simulink model "NaoLinearidadeAtuador"  (R2023b)
settings: Solver=FixedStepAuto  StartTime=0.0  StopTime=tf  FixedStep=step_modelo  RelTol=1e-3
values from neighbouring files (symbols this model uses):
  actuator_nonlin = inp.actuator_nonlin(i)    [RCS_Entradas.m]
  Td = inp.Td(i)    [RCS_Entradas.m]
  Tpulse = inp.Tpulse(i)    [RCS_Entradas.m]
settings Model: PacingRate=0.100000  Creator=rodri  LastModifiedBy=rodri
settings DataIOCC: SaveOutput=off  SaveTime=off

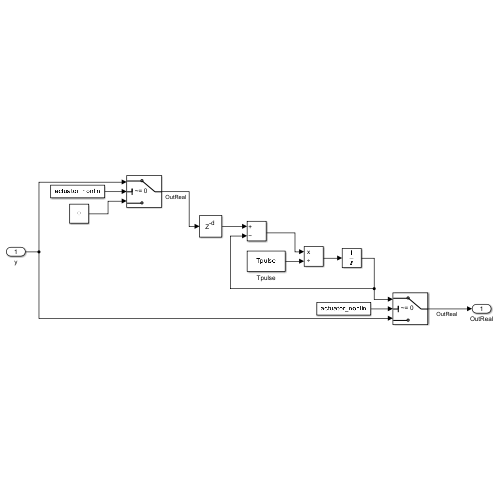
[thumbnail: Simulink's stored preview of the top-level diagram]
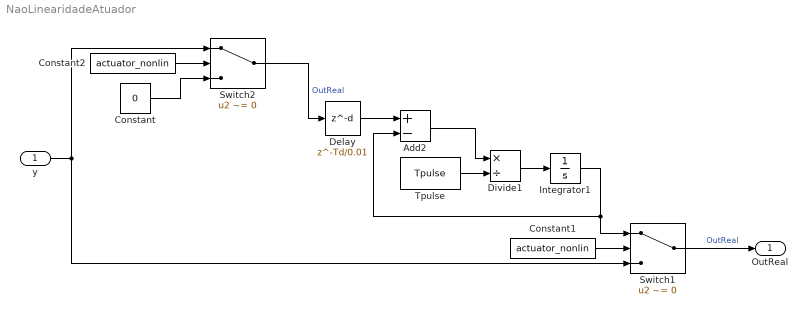
== system NaoLinearidadeAtuador ==
  y : Inport  OutDataTypeStr=double  PortDimensions=1
  Add2 : Sum  Inputs=+-
  Constant : Constant  Value=0
  Constant1 : Constant  Value=actuator_nonlin  OutDataTypeStr=boolean  SampleTime=-1
  Constant2 : Constant  Value=actuator_nonlin  OutDataTypeStr=boolean  SampleTime=-1
  Delay : Delay  DelayLength=Td/0.01  InitialCondition=0
  Divide1 : Product  Inputs=*/
  Integrator1 : Integrator
  Switch1 : Switch  Criteria=u2 ~= 0  SaturateOnIntegerOverflow=off  InputSameDT=off
  Switch2 : Switch  Criteria=u2 ~= 0  SaturateOnIntegerOverflow=off  InputSameDT=off
  Tpulse : Constant  Value=Tpulse  SampleTime=-1
  OutReal : Outport  OutDataTypeStr=double  PortDimensions=1  SampleTime=0
  wires:
  Switch1/1 -> OutReal/1  "OutReal"
  Constant1/1 -> Switch1/2
  Integrator1/1 -> Add2/2, Switch1/1
  Tpulse/1 -> Divide1/2
  Delay/1 -> Add2/1
  y/1 -> Switch1/3, Switch2/1
  Add2/1 -> Divide1/1
  Divide1/1 -> Integrator1/1
  Constant2/1 -> Switch2/2
  Switch2/1 -> Delay/1  "OutReal"
  Constant/1 -> Switch2/3
